simulink model "task4B_bc"  (R2024b)
settings: Solver=VariableStepAuto  StartTime=0.0  StopTime=4000  RelTol=1e-3
libraries: slctrl_linear x1
settings Model: Creator=brope  LastModifiedBy=brope

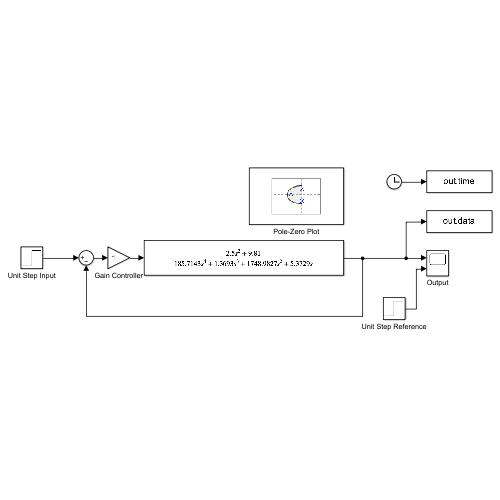
[thumbnail: Simulink's stored preview of the top-level diagram]
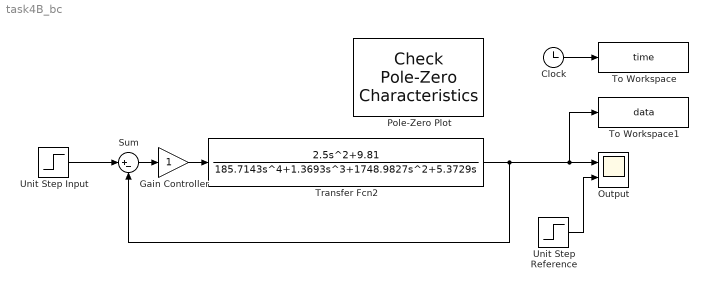
== system task4B_bc ==
  Clock : Clock
  Gain Controller : Gain
  Output : Scope  NumInputPorts=2
  Pole-Zero Plot : slctrl_linear/Check Pole-Zero Characteristics  InstantiateOnLoad=on  SaveOperatingPoints=off  LinearizationIOs={'/Gain Controller', 1, 'out', 'off', '';'/Unit Step Input', 1, 'in', 'off', ''}  LinearizeAt=SnapshotTimes  SnapshotTimes=[0]  TriggerType=rising  SampleTime=auto  RateConversionMethod=zoh  PreWarpFreq=10  UseExactDelayModel=off  UseFullBlockNameLabels=off  UseBusSignalLabels=off  enabled=on  stopWhenAssertionFail=off  export=off  ViewDlgPos=[1 49 1536 740.8]  LaunchViewOnOpen=on  OpenViewOnLoad=off  FrequencyUnits=rad/s  MagnitudeUnits=dB  PhaseUnits=deg  TimeUnits=seconds  EnableSettlingTime=off  SettlingTime=[]  EnablePercentOvershoot=off  PercentOvershoot=[]  EnableDampingRatio=off  DampingRatio=[]  EnableNaturalFrequency=off  NaturalFrequencyBound=>=  NaturalFrequency=[]
      settings: LibrarySourceBlock=slctrlblks/Linear Analysis Plots/Pole-Zero Plot  SaveToWorkspace=off  SaveName=sys
  Sum : Sum  Inputs=|+-
  To Workspace : ToWorkspace  VariableName=time
      settings: Save2DSignal=2-D array (concatenate along first dimension)
  To Workspace1 : ToWorkspace  VariableName=data
      settings: Save2DSignal=2-D array (concatenate along first dimension)
  Transfer Fcn2 : TransferFcn  Numerator=[2.5 0 9.81]  Denominator=[185.7143 1.3693 1748.9827 5.3729 0]  ParameterTunability=Optimized
  Unit Step Input : Step  SampleTime=0
  Unit Step Reference : Step  SampleTime=0
  wires:
  Unit Step Input/1 -> Sum/1
  Clock/1 -> To Workspace/1
  Unit Step Reference/1 -> Output/2
  Sum/1 -> Gain Controller/1
  Transfer Fcn2/1 -> To Workspace1/1, Output/1, Sum/2
  Gain Controller/1 -> Transfer Fcn2/1
